simulink model "questao2linearizadorelay"  (Simulink 6.0)
settings: Solver=ode45  StartTime=0.0  StopTime=10000.0  RelTol=1e-3
settings Model: Creator=usuario  LastModifiedBy=Thales Ruano
settings OptimizationCC: InlineInvariantSignals=off
settings DebuggingCC: SignalResolutionControl=UseLocalSettings
settings GRTTargetCC: TargetFcnLib=ansi_tfl_table_tmw.mat

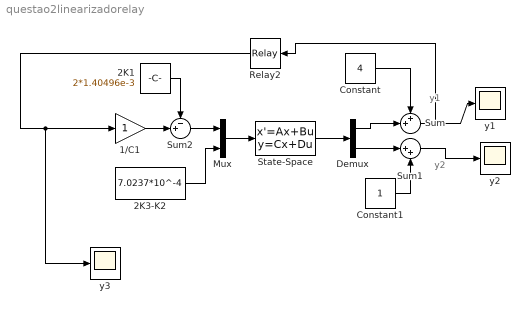
== system questao2linearizadorelay ==
  note: y1
  note: y2
  1/C1 : Gain
  2K1 : Constant  Value=2*1.40496e-3
  2K3-K2 : Constant  Value=7.0237*10^-4
  Constant : Constant  Value=4
  Constant1 : Constant
  Demux : Demux  Outputs=2
  Mux : Mux  Inputs=2
  Relay2 : Relay  Orientation=left  OnSwitchValue=5  OffSwitchValue=3  OnOutputValue=0  OffOutputValue=5e-3
  State-Space : StateSpace  A=[-0.25*1.404962946e-3 0;0.25*7.024814731e-4 -0.5*7.025918446e-4]  B=[1 0;0 1]  C=[1 0; 0 1]  D=[0 0;0 0]  X0=[0.5 -0.5]
  Sum : Sum  Inputs=++|
  Sum1 : Sum  Inputs=|++
  Sum2 : Sum  Inputs=-+|
  y1 : Scope
  y2 : Scope
  y3 : Scope
      settings: SaveName=ScopeData2
  wires:
  Demux/1 -> Sum/2
  Demux/2 -> Sum1/1
  State-Space/1 -> Demux/1
  Mux/1 -> State-Space/1
  Constant/1 -> Sum/1
  Constant1/1 -> Sum1/2
  2K3-K2/1 -> Mux/2
  Sum1/1 -> y2/1
  Sum/1 -> y1/1, Relay2/1
  1/C1/1 -> Sum2/2
  Sum2/1 -> Mux/1
  2K1/1 -> Sum2/1
  Relay2/1 -> 1/C1/1, y3/1
